simulink model "KF_Q_tempovariante"  (R2021a)
settings: Solver=ode45  StartTime=0.0  StopTime=tt(end)  MaxStep=0.1  RelTol=1e-3  EnableMultiTasking=on
model workspace (MATLAB code in the model file + MAT data in the model file):
  L = 2.5
  v0 = 0
  xe0 = 0
  xn0 = 0
  theta0 = 0
  Ts = 1
  rr = [0 0 0 0 0 0 0 0 0 0 0 0 ... (9404 elements, 9404x1)]
  tt = [0 0.05 0.1 0.15 0.2 0.25 0.3 0.35 0.4 0.45 0.5 0.55 ... (9404 elements, 9404x1)]
  vv = [25 25 25 25 25 25 25 25 25 25 25 25 ... (9404 elements, 9404x1)]
undefined symbols (not defined in the file or in its folder): Discrete, Time
libraries: simulink x4, pid_lib x2, ctrlSharedLib x1
(part 1 of 2)
settings Model: Creator=The MathWorks, Inc.  LastModifiedBy=angeloz
settings SolverCC: AlgebraicLoopSolver=TrustRegion
settings DataIOCC: SaveFormat=Array  SaveOutput=off  SignalLogging=off  DSMLogging=off  SaveTime=off  ReturnWorkspaceOutputs=off
settings OptimizationCC: LifeSpan=inf
settings DebuggingCC: AlgebraicLoopMsg=none  SolverPrmCheckMsg=warning  SFUnexpectedBacktrackingDiag=warning  SFNoUnconditionalDefaultTransitionDiag=warning  SFExecutionAtInitializationDiag=none  SFMachineParentedDataDiag=warning  ArithmeticOperatorsInVariantConditions=warning
settings HardwareCC: ProdBitPerPointer=32  ProdBitPerSizeT=32  ProdBitPerPtrDiffT=32  ProdLargestAtomicFloat=None  ProdIntDivRoundTo=Undefined  ProdEndianess=Unspecified  ProdWordSize=32  ProdHWDeviceType=32-bit Generic
settings ModelReferenceCC: PropagateSignalLabelsOutOfModel=off
settings SFSimCC: SimUseLocalCustomCode=off  CustomCodeUndefinedFunction=UseInterfaceOnly
settings RTWCC: RTWUseLocalCustomCode=off
settings CodeAppCC: StateflowObjectComments=on
settings GRTTargetCC: TargetLangStandard=C89/C90 (ANSI)
settings ConfigComp: CovMetricSettings=dw  CovSaveCumulativeToWorkspaceVar=on  CovSaveSingleToWorkspaceVar=on  CovExternalEMLEnable=off  CovSFcnEnable=off

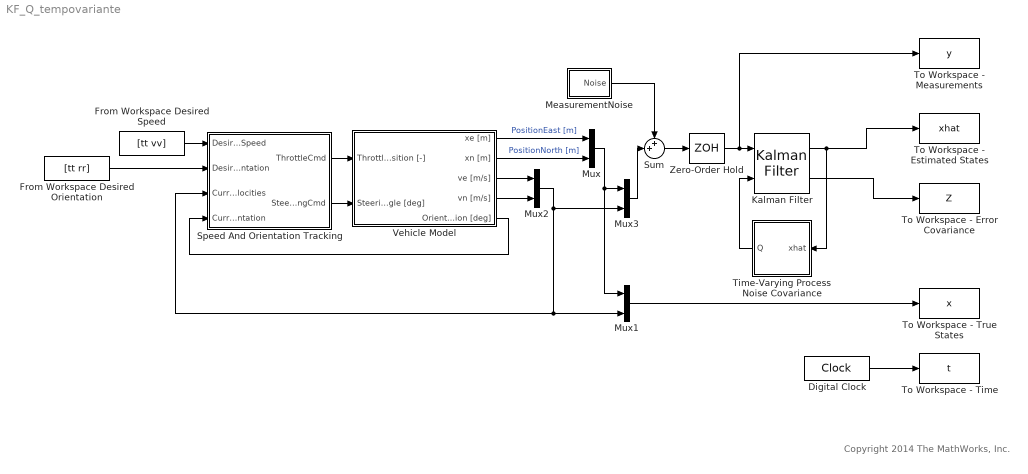
== system KF_Q_tempovariante ==
  note: Copyright 2014 The MathWorks, Inc.
  Digital Clock : DigitalClock  SampleTime=Ts
  From Workspace Desired Orientation : FromWorkspace  VariableName=[tt rr]
  From Workspace Desired Speed : FromWorkspace  VariableName=[tt vv]
  Kalman Filter : ctrlSharedLib/Kalman Filter  TimeDomain=Discrete-Time  UseCurrentEstimator=on  ModelSource=Individual A, B, C, D matrices  ModelSourceVariable=sys  A=[1 0 Ts 0; 0 1 0 Ts; 0 0 1 0; 0 0 0 1]  B=eye(2)  C=[1 0 0 0; 0 1 0 0; 0 0 1 0; 0 0 0 1]  D=zeros(2)  NumberOfStates=2  NumberOfInputs=2  NumberOfOutputs=2  InitialEstimateSource=Dialog  X0=0  P0=10  UseK=off  UseGH=on  NumberOfProcessNoiseInputs=2  G=[Ts/2 0; 0 Ts/2; 1 0; 0 1]  TimeInvariantG=on  H=0  TimeInvariantH=on  Q=0.05  TimeInvariantQ=off  R=50  TimeInvariantR=on  N=0  TimeInvariantN=on  AddInputPort=off  AddEnablePort=off  OutputEstimatedY=off  OutputP=on  Ts=Ts
  MeasurementNoise : Subsystem
  Mux{,1..3} (4 alike) : Mux  Inputs=2
  Speed And Orientation Tracking : Subsystem
  Sum : Sum  Inputs=++|
  Time-Varying Process Noise Covariance : Subsystem
  To Workspace - Error Covariance : ToWorkspace  VariableName=Z  SampleTime=-1
  To Workspace - Estimated States : ToWorkspace  VariableName=xhat  SampleTime=-1
      settings: Save2DSignal=2-D array (concatenate along first dimension)
  To Workspace - Measurements : ToWorkspace  VariableName=y  SampleTime=Ts
      settings: Save2DSignal=2-D array (concatenate along first dimension)
  To Workspace - Time : ToWorkspace  VariableName=t  SampleTime=-1
      settings: Save2DSignal=2-D array (concatenate along first dimension)
  To Workspace - True States : ToWorkspace  VariableName=x  SampleTime=Ts
      settings: Save2DSignal=2-D array (concatenate along first dimension)
  Vehicle Model : Subsystem
  Zero-Order Hold : ZeroOrderHold  SampleTime=Ts
  wires:
  Vehicle Model/2(xn [m]) -> Mux/2  "PositionNorth [m]"
  Mux1/1 -> To Workspace - True States/1
  Kalman Filter/1 -> Time-Varying Process Noise Covariance/1(xhat), To Workspace - Estimated States/1
  Vehicle Model/1(xe [m]) -> Mux/1  "PositionEast [m]"
  Digital Clock/1 -> To Workspace - Time/1
  Mux/1 -> Mux3/1, Mux1/1
  Sum/1 -> Zero-Order Hold/1
  MeasurementNoise/1(Noise) -> Sum/1
  Vehicle Model/4(vn [m/s]) -> Mux2/2
  Vehicle Model/3(ve [m/s]) -> Mux2/1
  Mux2/1 -> Mux3/2, Speed And Orientation Tracking/3(CurrentVelocities), Mux1/2
  Speed And Orientation Tracking/2(SteeringCmd) -> Vehicle Model/2("SteeringAngle [deg] ")
  Speed And Orientation Tracking/1(ThrottleCmd) -> Vehicle Model/1(ThrottlePosition [-])
  Vehicle Model/5(Orientation [deg]) -> Speed And Orientation Tracking/4(CurrentOrientation)
  From Workspace Desired Orientation/1 -> Speed And Orientation Tracking/2(DesiredOrientation)
  From Workspace Desired Speed/1 -> Speed And Orientation Tracking/1(DesiredSpeed)
  Time-Varying Process Noise Covariance/1(Q) -> Kalman Filter/2
  Kalman Filter/2 -> To Workspace - Error Covariance/1
  Zero-Order Hold/1 -> To Workspace - Measurements/1, Kalman Filter/1
  Mux3/1 -> Sum/2
